simulink model "Get_RE_Motor"  (R2013a)
settings: Solver=FixedStepDiscrete  StartTime=0.0  StopTime=60  RelTol=1e-3
undefined symbols (not defined in the file): Kd, Km, Ks, ts
libraries: arduino_io_lib x7, simulink x3
settings Model: Creator=cell  LastModifiedBy=cell
settings OptimizationCC: OptimizeModelRefInitCode=on  LifeSpan=1
settings DebuggingCC: StrictBusMsg=Warning
settings HardwareCC: ProdBitPerInt=16  ProdBitPerPointer=8  ProdIntDivRoundTo=Zero  ProdEndianess=LittleEndian  ProdWordSize=8  ProdHWDeviceType=Atmel->AVR
settings RTWCC: SystemTargetFile=realtime.tlc  GenerateMakefile=off  TemplateMakefile=realtime.tmf  Description=Run on Target Hardware  RTWVerbose=off  ProcessScript=realtime_make_rtw_hook
settings CodeAppCC: IgnoreCustomStorageClasses=off
settings STFCustomTargetCC: TargetLibSuffix=.a  GenerateSampleERTMain=on  CombineOutputUpdateFcns=on  ERTCustomFileBanners=on  SupportContinuousTime=off  SupportNonInlinedSFcns=off  MATLABClassNameForMDSCustomization=Simulink.SoftwareTarget.ERTCustomization  SystemTargetFile=realtime.tlc
settings ERTTargetCC: ParMdlRefBuildCompliant=off  CompOptLevelCompliant=off  ConcurrentExecutionCompliant=off  ERTFirstTimeCompliant=off  ModelStepFunctionPrototypeControlCompliant=off  CPPClassGenCompliant=off  ERTCustomFileTemplate=realtime_file_process.tlc

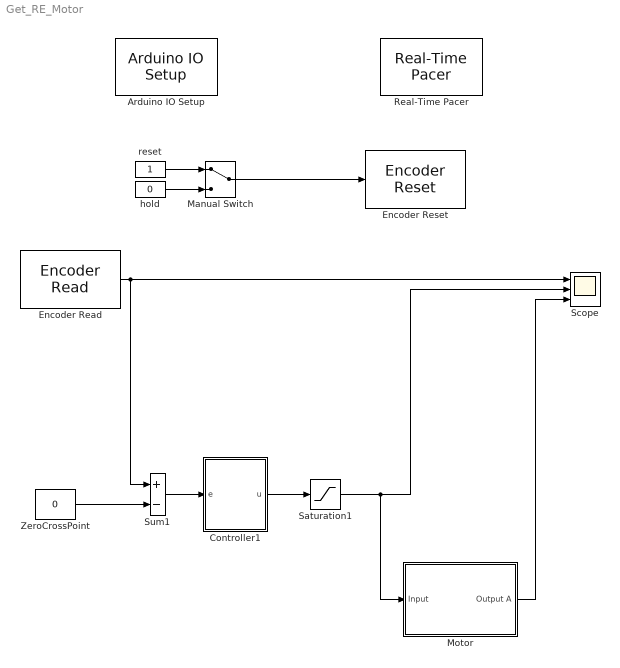
== system Get_RE_Motor ==
  " Controller1" : Subsystem
  Arduino IO Setup : arduino_io_lib/Arduino IO Setup  Priority=3  arduinoVar=Existing workspace arduino variable #1  workspaceVarName=a  comPort=DEMO
  Encoder Read : arduino_io_lib/Encoder Read  arduinoVar=Existing workspace arduino variable #1  encNum=1  pinA=2  pinB=3  DbDl=0  T=ts
  Encoder Reset : arduino_io_lib/Encoder Reset  arduinoVar=Existing workspace arduino variable #1  encNum=1  T=ts
  Manual Switch : ManualSwitch
  Motor : Subsystem
  Real-Time Pacer : arduino_io_lib/Real-Time Pacer  simTimePerRealTime=1
  Saturation1 : Saturate  UpperLimit=100  LowerLimit=-100
  Scope : Scope  NumInputPorts=3
      settings: TimeRange=10  YMin=-800~-100~0  YMax=600~100~3.75
  Sum1 : Sum  Inputs=+-
  ZeroCrossPoint : Constant  Value=0
  hold : Constant  Value=0
  reset : Constant
  wires:
  reset/1 -> Manual Switch/1
  hold/1 -> Manual Switch/2
  Manual Switch/1 -> Encoder Reset/1
  ZeroCrossPoint/1 -> Sum1/2
  Sum1/1 -> " Controller1"/1(e)
  Encoder Read/1 -> Scope/1, Sum1/1
  " Controller1"/1(u) -> Saturation1/1
  Saturation1/1 -> Motor/1(Input), Scope/2
  Motor/1(Output A) -> Scope/3

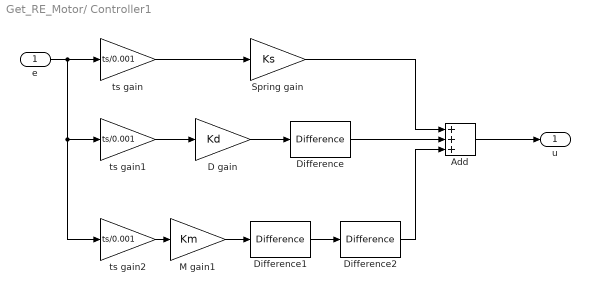
== system Get_RE_Motor/ Controller1 ==
  e : Inport
  Add : Sum  Inputs=+++
  D gain : Gain  Gain=Kd
  Difference : simulink/Discrete/Difference  ICPrevInput=0.0  InputProcessing=Inherited  OutMin=[]  OutMax=[]  OutDataType=fixdt(1, 16)  OutScaling=2^-10  DoSatur=off
  Difference1 : simulink/Discrete/Difference  ICPrevInput=0.0  InputProcessing=Inherited  OutMin=[]  OutMax=[]  OutDataType=fixdt(1, 16)  OutScaling=2^-10  DoSatur=off
  Difference2 : simulink/Discrete/Difference  ICPrevInput=0.0  InputProcessing=Inherited  OutMin=[]  OutMax=[]  OutDataType=fixdt(1, 16)  OutScaling=2^-10  DoSatur=off
  M gain1 : Gain  Gain=Km
  Spring gain : Gain  Gain=Ks
  ts gain : Gain  Gain=ts/0.001
  ts gain1 : Gain  Gain=ts/0.001
  ts gain2 : Gain  Gain=ts/0.001
  u : Outport
  wires:
  Spring gain/1 -> Add/1
  Add/1 -> u/1
  D gain/1 -> Difference/1
  Difference/1 -> Add/2
  e/1 -> ts gain/1, ts gain1/1, ts gain2/1
  M gain1/1 -> Difference1/1
  Difference2/1 -> Add/3
  Difference1/1 -> Difference2/1
  ts gain/1 -> Spring gain/1
  ts gain1/1 -> D gain/1
  ts gain2/1 -> M gain1/1

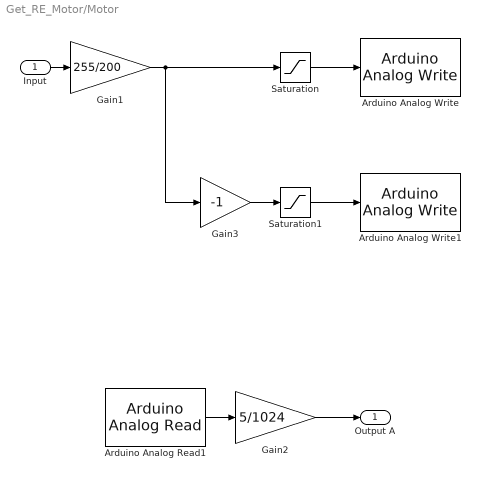
== system Get_RE_Motor/Motor ==
  Input : Inport
  Arduino Analog Read1 : arduino_io_lib/Arduino Analog Read  arduinoVar=Existing workspace arduino variable #1  arduinoPin=0  T=ts
  Arduino Analog Write : arduino_io_lib/Arduino Analog Write  arduinoVar=Existing workspace arduino variable #1  arduinoPin=5  T=ts
  Arduino Analog Write1 : arduino_io_lib/Arduino Analog Write  arduinoVar=Existing workspace arduino variable #1  arduinoPin=6  T=ts
  Gain1 : Gain  Gain=255/200
  Gain2 : Gain  Gain=5/1024
  Gain3 : Gain  Gain=-1
  Saturation : Saturate  UpperLimit=255  LowerLimit=0
  Saturation1 : Saturate  UpperLimit=255  LowerLimit=0
  Output A : Outport
  wires:
  Input/1 -> Gain1/1
  Arduino Analog Read1/1 -> Gain2/1
  Saturation/1 -> Arduino Analog Write/1
  Gain1/1 -> Gain3/1, Saturation/1
  Saturation1/1 -> Arduino Analog Write1/1
  Gain2/1 -> Output A/1
  Gain3/1 -> Saturation1/1
